simulink model "PmsmMotorCtrl"  (R2019b)
settings: Solver=VariableStepAuto  StartTime=0.0  StopTime=10  MaxStep=1E-3  RelTol=1e-3  EnableMultiTasking=on
model workspace (MAT data in the model file):
  Rs = 0
undefined symbols (not defined in the file or in its folder): J, k, Ld, Lq, N, PsiM, QCmdLim, QCmdRateLim
libraries: ElectricalModelLib x5, simulink x2
settings Model: OrderedModelArguments=off  Creator=The MathWorks, Inc.  LastModifiedBy=cleme
settings DataIOCC: LimitDataPoints=on  ReturnWorkspaceOutputs=off
settings OptimizationCC: LifeSpan=inf
settings DebuggingCC: AllowSymbolicDim=off  SFUnexpectedBacktrackingDiag=warning  SFNoUnconditionalDefaultTransitionDiag=warning  SFExecutionAtInitializationDiag=none  ArithmeticOperatorsInVariantConditions=warning
settings ModelReferenceCC: PropagateSignalLabelsOutOfModel=off
settings SFSimCC: SimUseLocalCustomCode=off  CustomCodeUndefinedFunction=UseInterfaceOnly
settings RTWCC: RTWUseLocalCustomCode=off
settings CodeAppCC: StateflowObjectComments=on
settings GRTTargetCC: TargetLangStandard=C89/C90 (ANSI)
settings ConfigComp: CovMetricSettings=dw  CovSaveCumulativeToWorkspaceVar=on  CovSaveSingleToWorkspaceVar=on  CovExternalEMLEnable=off

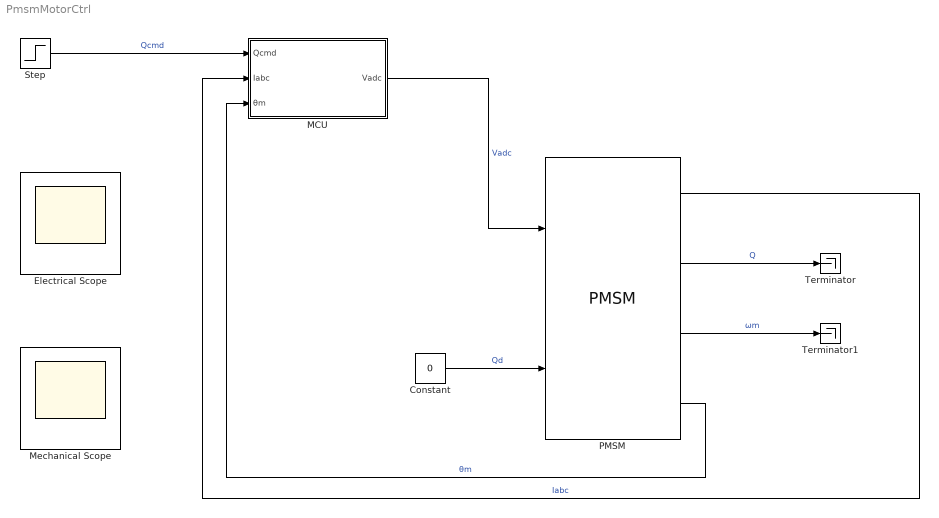
== system PmsmMotorCtrl ==
  Constant : Constant  Value=0
  Electrical Scope : Scope
      settings: Floating=on
  MCU : Subsystem
  Mechanical Scope : Scope
      settings: Floating=on
  PMSM : ElectricalModelLib/PMSM  N=N  Rs=Rs  Ld=Ld  Lq=Lq  L0=L0  PsiM=PsiM  J=J  k=k
      settings: SourceProductName=Electrical
  Step : Step  SampleTime=0
  Terminator : Terminator
  Terminator1 : Terminator
  wires:
  MCU/1(Vadc) -> PMSM/1  "Vadc"
  Constant/1 -> PMSM/2  "Qd"
  PMSM/1 -> MCU/2(Iabc)  "Iabc"
  PMSM/2 -> Terminator/1  "Q"
  PMSM/3 -> Terminator1/1  "ωm"
  PMSM/4 -> MCU/3(θm)  "θm"
  Step/1 -> MCU/1(Qcmd)  "Qcmd"

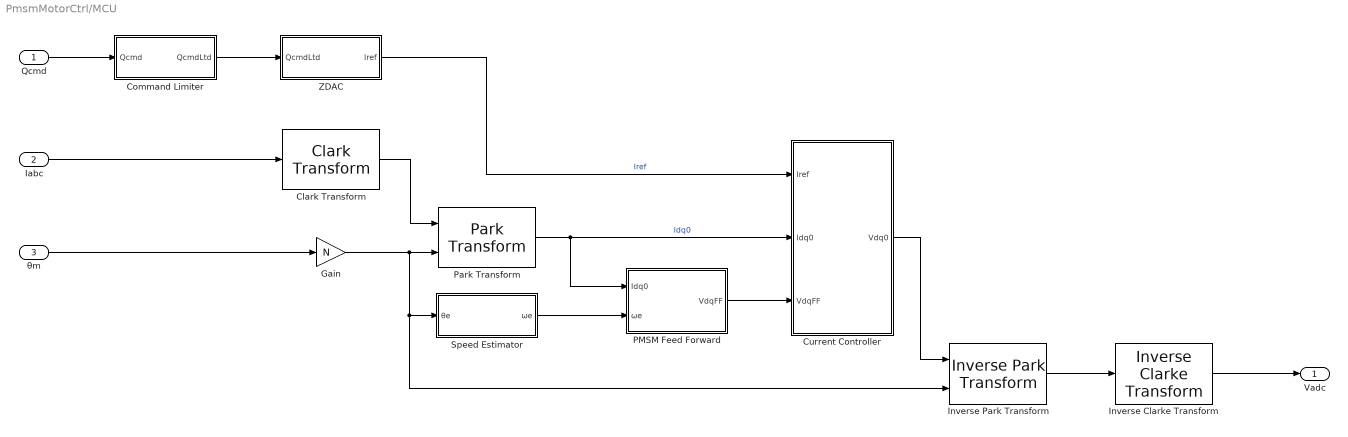
== system PmsmMotorCtrl/MCU ==
  Qcmd : Inport
  Iabc : Inport  Port=2
  θm : Inport  Port=3
  Clark Transform : ElectricalModelLib/Clark Transform
      settings: SourceProductName=Electrical
  Command Limiter : Subsystem
  Current Controller : Subsystem
  Gain : Gain  Gain=N
  Inverse Clarke Transform : ElectricalModelLib/Inverse Clarke Transform
      settings: SourceProductName=Electrical
  Inverse Park Transform : ElectricalModelLib/Inverse Park Transform
      settings: SourceProductName=Electrical
  PMSM Feed Forward : Subsystem
  Park Transform : ElectricalModelLib/Park Transform
      settings: SourceProductName=Electrical
  Speed Estimator : Subsystem
  ZDAC : Subsystem
  Vadc : Outport
  wires:
  θm/1 -> Gain/1
  Iabc/1 -> Clark Transform/1
  Clark Transform/1 -> Park Transform/1
  Gain/1 -> Speed Estimator/1(θe), Inverse Park Transform/2, Park Transform/2
  ZDAC/1(Iref) -> Current Controller/1(Iref)  "Iref"
  Park Transform/1 -> PMSM Feed Forward/1(Idq0), Current Controller/2(Idq0)  "Idq0"
  Current Controller/1(Vdq0) -> Inverse Park Transform/1
  Inverse Park Transform/1 -> Inverse Clarke Transform/1
  Inverse Clarke Transform/1 -> Vadc/1
  PMSM Feed Forward/1(VdqFF) -> Current Controller/3(VdqFF)
  Speed Estimator/1(ωe) -> PMSM Feed Forward/2(ωe)
  Qcmd/1 -> Command Limiter/1(Qcmd)
  Command Limiter/1(QcmdLtd) -> ZDAC/1(QcmdLtd)

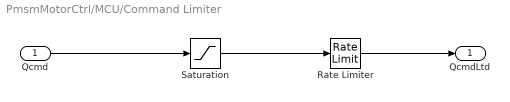
== system PmsmMotorCtrl/MCU/Command Limiter ==
  Qcmd : Inport
  Rate Limiter : RateLimiter  RisingSlewLimit=QCmdRateLim  FallingSlewLimit=-QCmdRateLim  SampleTimeMode=inherited
  Saturation : Saturate  UpperLimit=QCmdLim  LowerLimit=-QCmdLim
  QcmdLtd : Outport
  wires:
  Saturation/1 -> Rate Limiter/1
  Rate Limiter/1 -> QcmdLtd/1
  Qcmd/1 -> Saturation/1

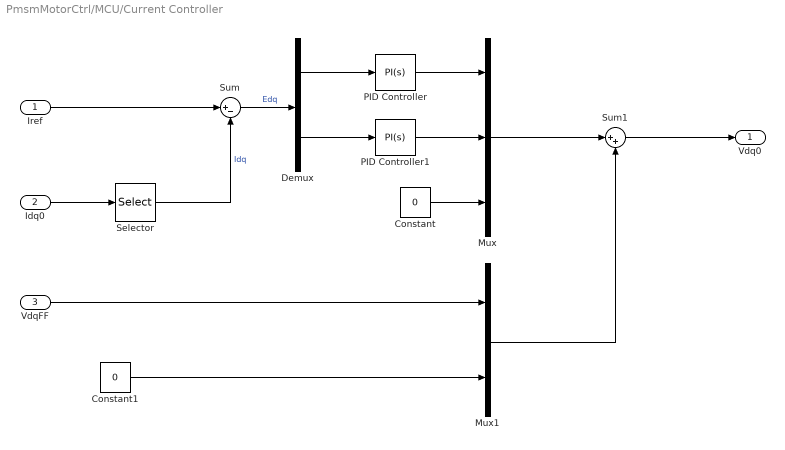
== system PmsmMotorCtrl/MCU/Current Controller ==
  Iref : Inport
  Idq0 : Inport  Port=2
  VdqFF : Inport  Port=3
  Constant : Constant  Value=0
  Constant1 : Constant  Value=0
  Demux : Demux  Outputs=2
  Mux : Mux  Inputs=3
  Mux1 : Mux  Inputs=2
  PID Controller : simulink/Continuous/PID Controller  Controller=PI  Form=Parallel  TimeDomain=Continuous-time  SampleTime=-1  IntegratorMethod=Forward Euler  FilterMethod=Forward Euler  ControllerParametersSource=internal  P=0.000190525588832577  I=0.00011  D=0  UseFilter=on  N=100  TunerSelectOption=Transfer Function Based (PID Tuner App)  InitialConditionSource=internal  InitialConditionForIntegrator=0  InitialConditionForFilter=0  DifferentiatorICPrevScaledInput=0  ExternalReset=none  TrackingMode=off  Kt=1  LimitOutput=off  UpperSaturationLimit=inf  LowerSaturationLimit=-inf  LinearizeAsGain=on  AntiWindupMode=none  Kb=1  POutMin=[]  POutMax=[]  IOutMin=[]  IOutMax=[]  DOutMin=[]  DOutMax=[]  NOutMin=[]  NOutMax=[]  SumOutMin=[]  SumOutMax=[]  SaturationOutMin=[]  SaturationOutMax=[]  PParamMin=[]  PParamMax=[]  IParamMin=[]  IParamMax=[]  DParamMin=[]  DParamMax=[]  NParamMin=[]  NParamMax=[]  KbParamMin=[]  KbParamMax=[]  KtParamMin=[]  KtParamMax=[]  KbOutMin=[]  KbOutMax=[]  KtOutMin=[]  KtOutMax=[]  IntegratorOutMin=[]  IntegratorOutMax=[]  FilterOutMin=[]  FilterOutMax=[]  SumI1OutMin=[]  SumI1OutMax=[]  SumI2OutMin=[]  SumI2OutMax=[]  SumI3OutMin=[]  SumI3OutMax=[]  SumI4OutMin=[]  SumI4OutMax=[]  SumDOutMin=[]  SumDOutMax=[]  DifferentiatorOutMin=[]  DifferentiatorOutMax=[]  FilterDiffOutCoefMin=[]  FilterDiffOutCoefMax=[]  ReciprocalOutMin=[]  ReciprocalOutMax=[]  SumDenOutMin=[]  SumDenOutMax=[]  SumNumOutMin=[]  SumNumOutMax=[]  DivideOutMin=[]  DivideOutMax=[]  IntegratorContinuousStateAttributes=''  IntegratorStateMustResolveToSignalObject=off  IntegratorRTWStateStorageClass=Auto  FilterContinuousStateAttributes=''  FilterStateMustResolveToSignalObject=off  FilterRTWStateStorageClass=Auto  ParallelPVariant=InternalParameters  IdealPVariant=Disabled  IVariant=InternalParameters  DVariant=Disabled  IntegratorVariant=Continuous  SatVariant=Disabled  AWVariant=Passthrough  PCopyVariant=Disabled  TRVariant=Disabled  FdbkBlocksVariant=Forward  IdealPFdbkVariant=Disabled  SatFdbkVariant=Disabled  DerivativeFilterVariant=Disabled  NVariant=Disabled  NCopyVariant=Disabled_SignalSpec  FilterICVariant=Disabled  IntegratorICVariant=InternalICs  ExternalResetVariant=Disabled  TRSumVariant=Passthrough  SumFdbkVariant=Disabled  SumVariant=Sum_PI
  PID Controller1 : simulink/Continuous/PID Controller  Controller=PI  Form=Parallel  TimeDomain=Continuous-time  SampleTime=-1  IntegratorMethod=Forward Euler  FilterMethod=Forward Euler  ControllerParametersSource=internal  P=0.323224704102505  I=319.000142447826  D=0  UseFilter=on  N=100  TunerSelectOption=Transfer Function Based (PID Tuner App)  InitialConditionSource=internal  InitialConditionForIntegrator=0  InitialConditionForFilter=0  DifferentiatorICPrevScaledInput=0  ExternalReset=none  TrackingMode=off  Kt=1  LimitOutput=off  UpperSaturationLimit=inf  LowerSaturationLimit=-inf  LinearizeAsGain=on  AntiWindupMode=none  Kb=1  POutMin=[]  POutMax=[]  IOutMin=[]  IOutMax=[]  DOutMin=[]  DOutMax=[]  NOutMin=[]  NOutMax=[]  SumOutMin=[]  SumOutMax=[]  SaturationOutMin=[]  SaturationOutMax=[]  PParamMin=[]  PParamMax=[]  IParamMin=[]  IParamMax=[]  DParamMin=[]  DParamMax=[]  NParamMin=[]  NParamMax=[]  KbParamMin=[]  KbParamMax=[]  KtParamMin=[]  KtParamMax=[]  KbOutMin=[]  KbOutMax=[]  KtOutMin=[]  KtOutMax=[]  IntegratorOutMin=[]  IntegratorOutMax=[]  FilterOutMin=[]  FilterOutMax=[]  SumI1OutMin=[]  SumI1OutMax=[]  SumI2OutMin=[]  SumI2OutMax=[]  SumI3OutMin=[]  SumI3OutMax=[]  SumI4OutMin=[]  SumI4OutMax=[]  SumDOutMin=[]  SumDOutMax=[]  DifferentiatorOutMin=[]  DifferentiatorOutMax=[]  FilterDiffOutCoefMin=[]  FilterDiffOutCoefMax=[]  ReciprocalOutMin=[]  ReciprocalOutMax=[]  SumDenOutMin=[]  SumDenOutMax=[]  SumNumOutMin=[]  SumNumOutMax=[]  DivideOutMin=[]  DivideOutMax=[]  IntegratorContinuousStateAttributes=''  IntegratorStateMustResolveToSignalObject=off  IntegratorRTWStateStorageClass=Auto  FilterContinuousStateAttributes=''  FilterStateMustResolveToSignalObject=off  FilterRTWStateStorageClass=Auto  ParallelPVariant=InternalParameters  IdealPVariant=Disabled  IVariant=InternalParameters  DVariant=Disabled  IntegratorVariant=Continuous  SatVariant=Disabled  AWVariant=Passthrough  PCopyVariant=Disabled  TRVariant=Disabled  FdbkBlocksVariant=Forward  IdealPFdbkVariant=Disabled  SatFdbkVariant=Disabled  DerivativeFilterVariant=Disabled  NVariant=Disabled  NCopyVariant=Disabled_SignalSpec  FilterICVariant=Disabled  IntegratorICVariant=InternalICs  ExternalResetVariant=Disabled  TRSumVariant=Passthrough  SumFdbkVariant=Disabled  SumVariant=Sum_PI
  Selector : Selector  InputPortWidth=3  IndexOptions=Index vector (dialog)  Indices=[1 2]  OutputSizes=1
  Sum : Sum  Inputs=|+-
  Sum1 : Sum  Inputs=|++
  Vdq0 : Outport
  wires:
  Sum1/1 -> Vdq0/1
  Idq0/1 -> Selector/1
  PID Controller1/1 -> Mux/2
  Demux/2 -> PID Controller1/1
  Demux/1 -> PID Controller/1
  Sum/1 -> Demux/1  "Edq"
  PID Controller/1 -> Mux/1
  Constant/1 -> Mux/3
  Iref/1 -> Sum/1
  Selector/1 -> Sum/2  "Idq"
  VdqFF/1 -> Mux1/1
  Constant1/1 -> Mux1/2
  Mux/1 -> Sum1/1
  Mux1/1 -> Sum1/2

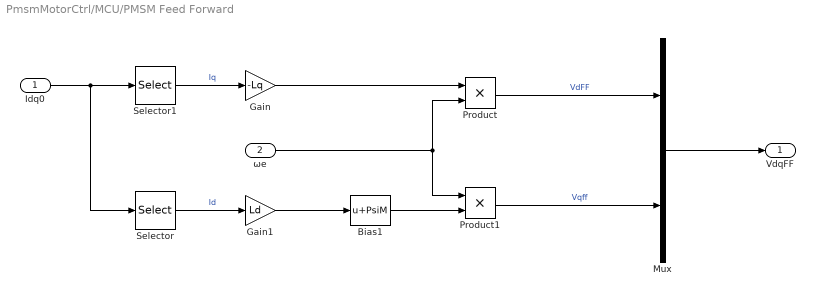
== system PmsmMotorCtrl/MCU/PMSM Feed Forward ==
  Idq0 : Inport
  ωe : Inport  Port=2
  Bias1 : Bias  Bias=PsiM
  Gain : Gain  Gain=-Lq
  Gain1 : Gain  Gain=Ld
  Mux : Mux  Inputs=2
  Product : Product
  Product1 : Product
  Selector : Selector  InputPortWidth=3  IndexOptions=Index vector (dialog)  Indices=1  OutputSizes=1
  Selector1 : Selector  InputPortWidth=3  IndexOptions=Index vector (dialog)  Indices=2  OutputSizes=1
  VdqFF : Outport
  wires:
  Idq0/1 -> Selector/1, Selector1/1
  Selector1/1 -> Gain/1  "Iq"
  Gain/1 -> Product/1
  ωe/1 -> Product1/1, Product/2
  Product/1 -> Mux/1  "VdFF"
  Gain1/1 -> Bias1/1
  Product1/1 -> Mux/2  "Vqff"
  Mux/1 -> VdqFF/1
  Bias1/1 -> Product1/2
  Selector/1 -> Gain1/1  "Id"

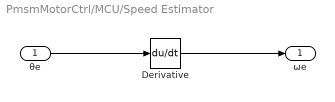
== system PmsmMotorCtrl/MCU/Speed Estimator ==
  θe : Inport
  Derivative : Derivative
  ωe : Outport
  wires:
  θe/1 -> Derivative/1
  Derivative/1 -> ωe/1

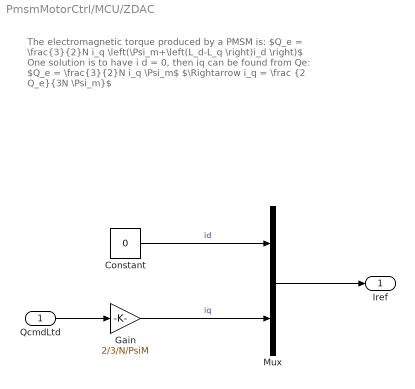
== system PmsmMotorCtrl/MCU/ZDAC ==
  note: The electromagnetic torque produced by a PMSM is:
      | $Q_e = \frac{3}{2}N i_q \left(\Psi_m+\left(L_d-L_q \right)i_d \right)$
      |
      | One solution is to have i d = 0, then iq can be found from Qe:
      | $Q_e = \frac{3}{2}N i_q \Psi_m$
      | $\Rightarrow i_q = \frac {2 Q_e}{3N \Psi_m}$
  QcmdLtd : Inport
  Constant : Constant  Value=0
  Gain : Gain  Gain=2/3/N/PsiM
      settings: AttributesFormatString=Gain = %<Gain>
  Mux : Mux  Inputs=2
  Iref : Outport
  wires:
  Mux/1 -> Iref/1
  QcmdLtd/1 -> Gain/1
  Constant/1 -> Mux/1  "id"
  Gain/1 -> Mux/2  "iq"
